simulink model "ThdRwLtStCalib"  (R2024b)
settings: Solver=FixedStepDiscrete  StartTime=0.0  StopTime=10.0  FixedStep=0.01  RelTol=1e-3
model workspace (MAT data in the model file):
  KeSMSwAcsMd6ThdRwLtStBkReclnUpwdDnwdPosMax_Val : Simulink.Parameter (value not decoded)
  KeSMSwAcsMd6ThdRwLtStBkReclnUpwdDnwdPosMin_Val : Simulink.Parameter (value not decoded)
  KeSMSwAcsMd6ThdRwLtStBkReclnUpwdDnwdPos_Val : Simulink.Parameter (value not decoded)
  KeSMSwAcsMd6ThdRwLtStCshnFldUpwdDnwdPosMax_Val : Simulink.Parameter (value not decoded)
  KeSMSwAcsMd6ThdRwLtStCshnFldUpwdDnwdPosMin_Val : Simulink.Parameter (value not decoded)
  KeSMSwAcsMd6ThdRwLtStCshnFldUpwdDnwdPos_Val : Simulink.Parameter (value not decoded)
  KeSMSwAcsMd6ThdRwLtStFrwdBkwdPosMax_Val : Simulink.Parameter (value not decoded)
  KeSMSwAcsMd6ThdRwLtStFrwdBkwdPosMin_Val : Simulink.Parameter (value not decoded)
  KeSMSwAcsMd6ThdRwLtStFrwdBkwdPos_Val : Simulink.Parameter (value not decoded)
symbols that are objects in the model workspace (value not decoded): KeSMSwAcsMd6ThdRwLtStBkReclnUpwdDnwdPos_Val, KeSMSwAcsMd6ThdRwLtStBkReclnUpwdDnwdPosMax_Val, KeSMSwAcsMd6ThdRwLtStBkReclnUpwdDnwdPosMin_Val, KeSMSwAcsMd6ThdRwLtStCshnFldUpwdDnwdPos_Val, KeSMSwAcsMd6ThdRwLtStCshnFldUpwdDnwdPosMax_Val, KeSMSwAcsMd6ThdRwLtStCshnFldUpwdDnwdPosMin_Val, KeSMSwAcsMd6ThdRwLtStFrwdBkwdPos_Val, KeSMSwAcsMd6ThdRwLtStFrwdBkwdPosMax_Val, KeSMSwAcsMd6ThdRwLtStFrwdBkwdPosMin_Val
undefined symbols (not defined in the file or in its folder): KeSMSw6sAcsEntryThdRwLtStBkReclnUpwdDnwdPos_Val, KeSMSw6sAcsEntryThdRwLtStBkReclnUpwdDnwdPosMax_Val, KeSMSw6sAcsEntryThdRwLtStBkReclnUpwdDnwdPosMin_Val, KeSMSw6sAcsEntryThdRwLtStCshnFldUpwdDnwdPos_Val, KeSMSw6sAcsEntryThdRwLtStCshnFldUpwdDnwdPosMax_Val, KeSMSw6sAcsEntryThdRwLtStCshnFldUpwdDnwdPosMin_Val, KeSMSw6sAcsEntryThdRwLtStFrwdBkwdPos_Val, KeSMSw6sAcsEntryThdRwLtStFrwdBkwdPosMax_Val, KeSMSw6sAcsEntryThdRwLtStFrwdBkwdPosMin_Val, KeSMSw6SAcsMd56ThdRwLtStBkReclnUpwdDnwdPos_Val, KeSMSw6SAcsMd56ThdRwLtStBkReclnUpwdDnwdPosMax_Val, KeSMSw6SAcsMd56ThdRwLtStBkReclnUpwdDnwdPosMin_Val, KeSMSw6SAcsMd56ThdRwLtStFrwdBkwdPos_Val, KeSMSw6SAcsMd56ThdRwLtStFrwdBkwdPosMax_Val, KeSMSw6SAcsMd56ThdRwLtStFrwdBkwdPosMin_Val, KeSMSw6sFamilyLMdThdRwLtStFrwdBkwdPos_Val, KeSMSw6sFamilyLMdThdRwLtStFrwdBkwdPosMax_Val, KeSMSw6sFamilyLMdThdRwLtStFrwdBkwdPosMin_Val, KeSMSw6sFamilyMdThdRwLtStFrwdBkwdPos_Val, KeSMSw6sFamilyMdThdRwLtStFrwdBkwdPosMax_Val, KeSMSw6sFamilyMdThdRwLtStFrwdBkwdPosMin_Val, KeSMSw6sLugThdRwLtStBkReclnUpwdDnwdPos_Val, KeSMSw6sLugThdRwLtStBkReclnUpwdDnwdPosMax_Val, KeSMSw6sLugThdRwLtStBkReclnUpwdDnwdPosMin_Val, KeSMSw6sLugThdRwLtStCshnFldUpwdDnwdPos_Val, KeSMSw6sLugThdRwLtStCshnFldUpwdDnwdPosMax_Val, KeSMSw6sLugThdRwLtStCshnFldUpwdDnwdPosMin_Val, KeSMSw6sVIPThdRwLtStBkReclnUpwdDnwdPos_Val, KeSMSw6sVIPThdRwLtStBkReclnUpwdDnwdPosMax_Val, KeSMSw6sVIPThdRwLtStBkReclnUpwdDnwdPosMin_Val, KeSMSw6sVIPThdRwLtStFrwdBkwdPos_Val, KeSMSw6sVIPThdRwLtStFrwdBkwdPosMax_Val, KeSMSw6sVIPThdRwLtStFrwdBkwdPosMin_Val, KeSMSwAcsEntryThdRwLtStBkReclnUpwdDnwdPos_Val, KeSMSwAcsEntryThdRwLtStBkReclnUpwdDnwdPosMax_Val, KeSMSwAcsEntryThdRwLtStBkReclnUpwdDnwdPosMin_Val, KeSMSwAcsEntryThdRwLtStCshnFldUpwdDnwdPos_Val, KeSMSwAcsEntryThdRwLtStCshnFldUpwdDnwdPosMax_Val, KeSMSwAcsEntryThdRwLtStCshnFldUpwdDnwdPosMin_Val, KeSMSwAcsEntryThdRwLtStFrwdBkwdPos_Val, KeSMSwAcsEntryThdRwLtStFrwdBkwdPosMax_Val, KeSMSwAcsEntryThdRwLtStFrwdBkwdPosMin_Val, KeSMSwAcsMd32ThdRwLtBkReclnUpwdDnwdPos_Val, KeSMSwAcsMd32ThdRwLtBkReclnUpwdDnwdPosMax_Val, KeSMSwAcsMd32ThdRwLtBkReclnUpwdDnwdPosMin_Val, KeSMSwAcsMd32ThdRwLtFldUpwdDnwdPos_Val, KeSMSwAcsMd32ThdRwLtFldUpwdDnwdPosMax_Val, KeSMSwAcsMd32ThdRwLtFldUpwdDnwdPosMin_Val, KeSMSwAcsMd56ThdRwLtStBkReclnUpwdDnwdPos_Val, KeSMSwAcsMd56ThdRwLtStBkReclnUpwdDnwdPosMax_Val, KeSMSwAcsMd56ThdRwLtStBkReclnUpwdDnwdPosMin_Val, KeSMSwAcsMd56ThdRwLtStCshnFldUpwdDnwdPos_Val, KeSMSwAcsMd56ThdRwLtStCshnFldUpwdDnwdPosMax_Val, KeSMSwAcsMd56ThdRwLtStCshnFldUpwdDnwdPosMin_Val, KeSMSwAcsMd56ThdRwLtStFrwdBkwdPos_Val, KeSMSwAcsMd56ThdRwLtStFrwdBkwdPosMax_Val, KeSMSwAcsMd56ThdRwLtStFrwdBkwdPosMin_Val, KeSMSwAcsMd57ThdRwLtStBkReclnUpwdDnwdPos_Val, KeSMSwAcsMd57ThdRwLtStBkReclnUpwdDnwdPosMax_Val, KeSMSwAcsMd57ThdRwLtStBkReclnUpwdDnwdPosMin_Val ... (+28)
libraries: TrgtPosSelcLib x20
(part 2 of 2)

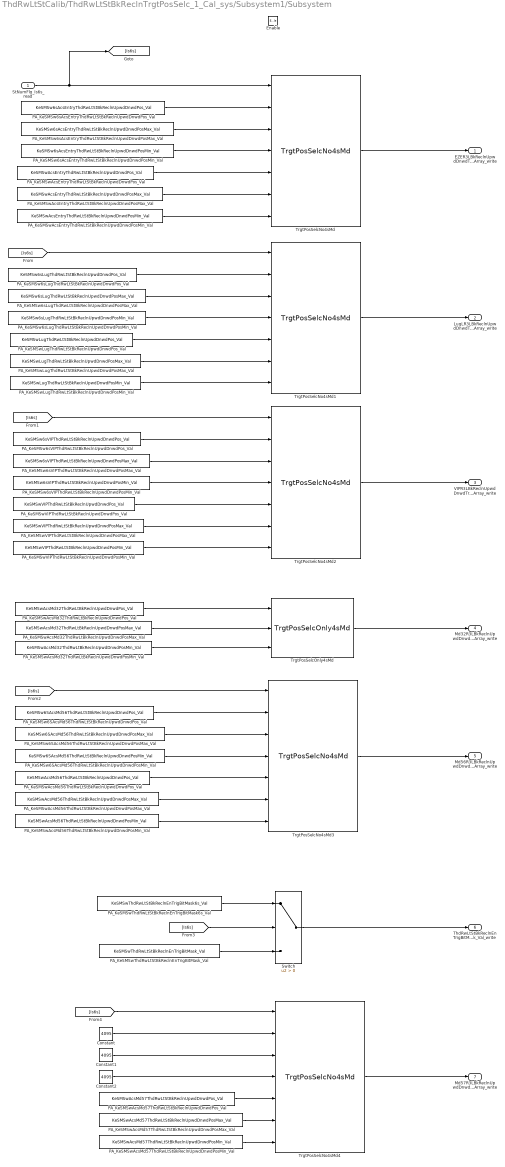
== system ThdRwLtStCalib/ThdRwLtStBkReclnTrgtPosSelc_1_Cal_sys/Subsystem1/Subsystem ==
  StNumFlg_Is6s_read : Inport
  Enable : EnablePort
  Constant : Constant  Value=4095  OutDataTypeStr=uint16
  Constant1 : Constant  Value=4095  OutDataTypeStr=uint16
  Constant2 : Constant  Value=4095  OutDataTypeStr=uint16
  PA_KeSMSw6SAcsMd56ThdRwLtStBkReclnUpwdDnwdPosMax_Val : Constant  Value=KeSMSw6SAcsMd56ThdRwLtStBkReclnUpwdDnwdPosMax_Val
  PA_KeSMSw6SAcsMd56ThdRwLtStBkReclnUpwdDnwdPosMin_Val : Constant  Value=KeSMSw6SAcsMd56ThdRwLtStBkReclnUpwdDnwdPosMin_Val
  PA_KeSMSw6SAcsMd56ThdRwLtStBkReclnUpwdDnwdPos_Val : Constant  Value=KeSMSw6SAcsMd56ThdRwLtStBkReclnUpwdDnwdPos_Val
  PA_KeSMSw6sAcsEntryThdRwLtStBkReclnUpwdDnwdPosMax_Val : Constant  Value=KeSMSw6sAcsEntryThdRwLtStBkReclnUpwdDnwdPosMax_Val
  PA_KeSMSw6sAcsEntryThdRwLtStBkReclnUpwdDnwdPosMin_Val : Constant  Value=KeSMSw6sAcsEntryThdRwLtStBkReclnUpwdDnwdPosMin_Val
  PA_KeSMSw6sAcsEntryThdRwLtStBkReclnUpwdDnwdPos_Val : Constant  Value=KeSMSw6sAcsEntryThdRwLtStBkReclnUpwdDnwdPos_Val
  PA_KeSMSw6sLugThdRwLtStBkReclnUpwdDnwdPosMax_Val : Constant  Value=KeSMSw6sLugThdRwLtStBkReclnUpwdDnwdPosMax_Val
  PA_KeSMSw6sLugThdRwLtStBkReclnUpwdDnwdPosMin_Val : Constant  Value=KeSMSw6sLugThdRwLtStBkReclnUpwdDnwdPosMin_Val
  PA_KeSMSw6sLugThdRwLtStBkReclnUpwdDnwdPos_Val : Constant  Value=KeSMSw6sLugThdRwLtStBkReclnUpwdDnwdPos_Val
  PA_KeSMSw6sVIPThdRwLtStBkReclnUpwdDnwdPosMax_Val : Constant  Value=KeSMSw6sVIPThdRwLtStBkReclnUpwdDnwdPosMax_Val
  PA_KeSMSw6sVIPThdRwLtStBkReclnUpwdDnwdPosMin_Val : Constant  Value=KeSMSw6sVIPThdRwLtStBkReclnUpwdDnwdPosMin_Val
  PA_KeSMSw6sVIPThdRwLtStBkReclnUpwdDnwdPos_Val : Constant  Value=KeSMSw6sVIPThdRwLtStBkReclnUpwdDnwdPos_Val
  PA_KeSMSwAcsEntryThdRwLtStBkReclnUpwdDnwdPosMax_Val : Constant  Value=KeSMSwAcsEntryThdRwLtStBkReclnUpwdDnwdPosMax_Val
  PA_KeSMSwAcsEntryThdRwLtStBkReclnUpwdDnwdPosMin_Val : Constant  Value=KeSMSwAcsEntryThdRwLtStBkReclnUpwdDnwdPosMin_Val
  PA_KeSMSwAcsEntryThdRwLtStBkReclnUpwdDnwdPos_Val : Constant  Value=KeSMSwAcsEntryThdRwLtStBkReclnUpwdDnwdPos_Val
  PA_KeSMSwAcsMd32ThdRwLtBkReclnUpwdDnwdPosMax_Val : Constant  Value=KeSMSwAcsMd32ThdRwLtBkReclnUpwdDnwdPosMax_Val
  PA_KeSMSwAcsMd32ThdRwLtBkReclnUpwdDnwdPosMin_Val : Constant  Value=KeSMSwAcsMd32ThdRwLtBkReclnUpwdDnwdPosMin_Val
  PA_KeSMSwAcsMd32ThdRwLtBkReclnUpwdDnwdPos_Val : Constant  Value=KeSMSwAcsMd32ThdRwLtBkReclnUpwdDnwdPos_Val
  PA_KeSMSwAcsMd56ThdRwLtStBkReclnUpwdDnwdPosMax_Val : Constant  Value=KeSMSwAcsMd56ThdRwLtStBkReclnUpwdDnwdPosMax_Val
  PA_KeSMSwAcsMd56ThdRwLtStBkReclnUpwdDnwdPosMin_Val : Constant  Value=KeSMSwAcsMd56ThdRwLtStBkReclnUpwdDnwdPosMin_Val
  PA_KeSMSwAcsMd56ThdRwLtStBkReclnUpwdDnwdPos_Val : Constant  Value=KeSMSwAcsMd56ThdRwLtStBkReclnUpwdDnwdPos_Val
  PA_KeSMSwAcsMd57ThdRwLtStBkReclnUpwdDnwdPosMax_Val : Constant  Value=KeSMSwAcsMd57ThdRwLtStBkReclnUpwdDnwdPosMax_Val
  PA_KeSMSwAcsMd57ThdRwLtStBkReclnUpwdDnwdPosMin_Val : Constant  Value=KeSMSwAcsMd57ThdRwLtStBkReclnUpwdDnwdPosMin_Val
  PA_KeSMSwAcsMd57ThdRwLtStBkReclnUpwdDnwdPos_Val : Constant  Value=KeSMSwAcsMd57ThdRwLtStBkReclnUpwdDnwdPos_Val
  PA_KeSMSwLugThdRwLtStBkReclnUpwdDnwdPosMax_Val : Constant  Value=KeSMSwLugThdRwLtStBkReclnUpwdDnwdPosMax_Val
  PA_KeSMSwLugThdRwLtStBkReclnUpwdDnwdPosMin_Val : Constant  Value=KeSMSwLugThdRwLtStBkReclnUpwdDnwdPosMin_Val
  PA_KeSMSwLugThdRwLtStBkReclnUpwdDnwdPos_Val : Constant  Value=KeSMSwLugThdRwLtStBkReclnUpwdDnwdPos_Val
  PA_KeSMSwThdRwLtStBkReclnEnTrigBitMask6s_Val : Constant  Value=KeSMSwThdRwLtStBkReclnEnTrigBitMask6s_Val
  PA_KeSMSwThdRwLtStBkReclnEnTrigBitMask_Val : Constant  Value=KeSMSwThdRwLtStBkReclnEnTrigBitMask_Val
  PA_KeSMSwVIPThdRwLtStBkReclnUpwdDnwdPosMax_Val : Constant  Value=KeSMSwVIPThdRwLtStBkReclnUpwdDnwdPosMax_Val
  PA_KeSMSwVIPThdRwLtStBkReclnUpwdDnwdPosMin_Val : Constant  Value=KeSMSwVIPThdRwLtStBkReclnUpwdDnwdPosMin_Val
  PA_KeSMSwVIPThdRwLtStBkReclnUpwdDnwdPos_Val : Constant  Value=KeSMSwVIPThdRwLtStBkReclnUpwdDnwdPos_Val
  Switch : Switch  Criteria=u2 > Threshold  SaturateOnIntegerOverflow=off  InputSameDT=off
  TrgtPosSelcNo4sMd{,1..4} (5 alike) : TrgtPosSelcLib/TrgtPosSelcNo4sMd  SystemSampleTime=-1  VariantActivationTime=update diagram  AllowFlexibleInterface=on  Latency=0  AutoFrameSizeCalculation=off
  TrgtPosSelcOnly4sMd : TrgtPosSelcLib/TrgtPosSelcOnly4sMd  SystemSampleTime=-1  VariantActivationTime=update diagram  AllowFlexibleInterface=on  Latency=0  AutoFrameSizeCalculation=off
  EZER3LBkReclnUpwdDnwdTrgtPosCalib_TrgtPosArray_write : Outport  VectorParamsAs1DForOutWhenUnconnected=off
      settings: EnsureOutportIsVirtual=on
  LugLR3LBkReclnUpwdDnwdTrgtPosCalib_TrgtPosArray_write : Outport  Port=2  VectorParamsAs1DForOutWhenUnconnected=off
      settings: EnsureOutportIsVirtual=on
  VIPR3LBkReclnUpwdDnwdTrgtPosCalib_TrgtPosArray_write : Outport  Port=3  VectorParamsAs1DForOutWhenUnconnected=off
      settings: EnsureOutportIsVirtual=on
  Md32R3LBkReclnUpwdDnwdTrgtPosCalib_TrgtPosArray_write : Outport  Port=4  VectorParamsAs1DForOutWhenUnconnected=off
      settings: EnsureOutportIsVirtual=on
  Md56R3LBkReclnUpwdDnwdTrgtPosCalib_TrgtPosArray_write : Outport  Port=5  VectorParamsAs1DForOutWhenUnconnected=off
      settings: EnsureOutportIsVirtual=on
  ThdRwLtStBkReclnEnTrigBitMask_Val_write : Outport  Port=6  VectorParamsAs1DForOutWhenUnconnected=off
      settings: EnsureOutportIsVirtual=on
  Md57R3LBkReclnUpwdDnwdTrgtPosCalib_TrgtPosArray_write : Outport  Port=7  VectorParamsAs1DForOutWhenUnconnected=off
      settings: EnsureOutportIsVirtual=on
  wires:
  StNumFlg_Is6s_read/1 -> [Is6s], TrgtPosSelcNo4sMd/1
  TrgtPosSelcNo4sMd1/1 -> LugLR3LBkReclnUpwdDnwdTrgtPosCalib_TrgtPosArray_write/1
  TrgtPosSelcNo4sMd2/1 -> VIPR3LBkReclnUpwdDnwdTrgtPosCalib_TrgtPosArray_write/1
  TrgtPosSelcNo4sMd/1 -> EZER3LBkReclnUpwdDnwdTrgtPosCalib_TrgtPosArray_write/1
  [Is6s] -> TrgtPosSelcNo4sMd1/1
  PA_KeSMSw6sAcsEntryThdRwLtStBkReclnUpwdDnwdPosMax_Val/1 -> TrgtPosSelcNo4sMd/3
  PA_KeSMSw6sAcsEntryThdRwLtStBkReclnUpwdDnwdPosMin_Val/1 -> TrgtPosSelcNo4sMd/4
  PA_KeSMSw6sAcsEntryThdRwLtStBkReclnUpwdDnwdPos_Val/1 -> TrgtPosSelcNo4sMd/2
  PA_KeSMSw6sLugThdRwLtStBkReclnUpwdDnwdPosMax_Val/1 -> TrgtPosSelcNo4sMd1/3
  PA_KeSMSw6sLugThdRwLtStBkReclnUpwdDnwdPos_Val/1 -> TrgtPosSelcNo4sMd1/2
  PA_KeSMSw6sLugThdRwLtStBkReclnUpwdDnwdPosMin_Val/1 -> TrgtPosSelcNo4sMd1/4
  [Is6s] -> TrgtPosSelcNo4sMd2/1
  PA_KeSMSw6sVIPThdRwLtStBkReclnUpwdDnwdPosMax_Val/1 -> TrgtPosSelcNo4sMd2/3
  PA_KeSMSw6sVIPThdRwLtStBkReclnUpwdDnwdPos_Val/1 -> TrgtPosSelcNo4sMd2/2
  PA_KeSMSw6sVIPThdRwLtStBkReclnUpwdDnwdPosMin_Val/1 -> TrgtPosSelcNo4sMd2/4
  PA_KeSMSwAcsEntryThdRwLtStBkReclnUpwdDnwdPosMax_Val/1 -> TrgtPosSelcNo4sMd/6
  PA_KeSMSwAcsEntryThdRwLtStBkReclnUpwdDnwdPosMin_Val/1 -> TrgtPosSelcNo4sMd/7
  PA_KeSMSwAcsEntryThdRwLtStBkReclnUpwdDnwdPos_Val/1 -> TrgtPosSelcNo4sMd/5
  PA_KeSMSwLugThdRwLtStBkReclnUpwdDnwdPosMax_Val/1 -> TrgtPosSelcNo4sMd1/6
  PA_KeSMSwLugThdRwLtStBkReclnUpwdDnwdPosMin_Val/1 -> TrgtPosSelcNo4sMd1/7
  PA_KeSMSwLugThdRwLtStBkReclnUpwdDnwdPos_Val/1 -> TrgtPosSelcNo4sMd1/5
  PA_KeSMSwVIPThdRwLtStBkReclnUpwdDnwdPosMax_Val/1 -> TrgtPosSelcNo4sMd2/6
  PA_KeSMSwVIPThdRwLtStBkReclnUpwdDnwdPos_Val/1 -> TrgtPosSelcNo4sMd2/5
  PA_KeSMSwVIPThdRwLtStBkReclnUpwdDnwdPosMin_Val/1 -> TrgtPosSelcNo4sMd2/7
  PA_KeSMSwAcsMd32ThdRwLtBkReclnUpwdDnwdPosMin_Val/1 -> TrgtPosSelcOnly4sMd/3
  PA_KeSMSwAcsMd32ThdRwLtBkReclnUpwdDnwdPosMax_Val/1 -> TrgtPosSelcOnly4sMd/2
  PA_KeSMSwAcsMd32ThdRwLtBkReclnUpwdDnwdPos_Val/1 -> TrgtPosSelcOnly4sMd/1
  TrgtPosSelcOnly4sMd/1 -> Md32R3LBkReclnUpwdDnwdTrgtPosCalib_TrgtPosArray_write/1
  [Is6s] -> TrgtPosSelcNo4sMd3/1
  PA_KeSMSw6SAcsMd56ThdRwLtStBkReclnUpwdDnwdPos_Val/1 -> TrgtPosSelcNo4sMd3/2
  PA_KeSMSw6SAcsMd56ThdRwLtStBkReclnUpwdDnwdPosMax_Val/1 -> TrgtPosSelcNo4sMd3/3
  PA_KeSMSw6SAcsMd56ThdRwLtStBkReclnUpwdDnwdPosMin_Val/1 -> TrgtPosSelcNo4sMd3/4
  PA_KeSMSwAcsMd56ThdRwLtStBkReclnUpwdDnwdPos_Val/1 -> TrgtPosSelcNo4sMd3/5
  PA_KeSMSwAcsMd56ThdRwLtStBkReclnUpwdDnwdPosMax_Val/1 -> TrgtPosSelcNo4sMd3/6
  PA_KeSMSwAcsMd56ThdRwLtStBkReclnUpwdDnwdPosMin_Val/1 -> TrgtPosSelcNo4sMd3/7
  TrgtPosSelcNo4sMd3/1 -> Md56R3LBkReclnUpwdDnwdTrgtPosCalib_TrgtPosArray_write/1
  PA_KeSMSwThdRwLtStBkReclnEnTrigBitMask6s_Val/1 -> Switch/1
  [Is6s] -> Switch/2
  PA_KeSMSwThdRwLtStBkReclnEnTrigBitMask_Val/1 -> Switch/3
  Switch/1 -> ThdRwLtStBkReclnEnTrigBitMask_Val_write/1
  [Is6s] -> TrgtPosSelcNo4sMd4/1
  PA_KeSMSwAcsMd57ThdRwLtStBkReclnUpwdDnwdPos_Val/1 -> TrgtPosSelcNo4sMd4/5
  PA_KeSMSwAcsMd57ThdRwLtStBkReclnUpwdDnwdPosMax_Val/1 -> TrgtPosSelcNo4sMd4/6
  PA_KeSMSwAcsMd57ThdRwLtStBkReclnUpwdDnwdPosMin_Val/1 -> TrgtPosSelcNo4sMd4/7
  Constant/1 -> TrgtPosSelcNo4sMd4/2
  Constant1/1 -> TrgtPosSelcNo4sMd4/3
  Constant2/1 -> TrgtPosSelcNo4sMd4/4
  TrgtPosSelcNo4sMd4/1 -> Md57R3LBkReclnUpwdDnwdTrgtPosCalib_TrgtPosArray_write/1

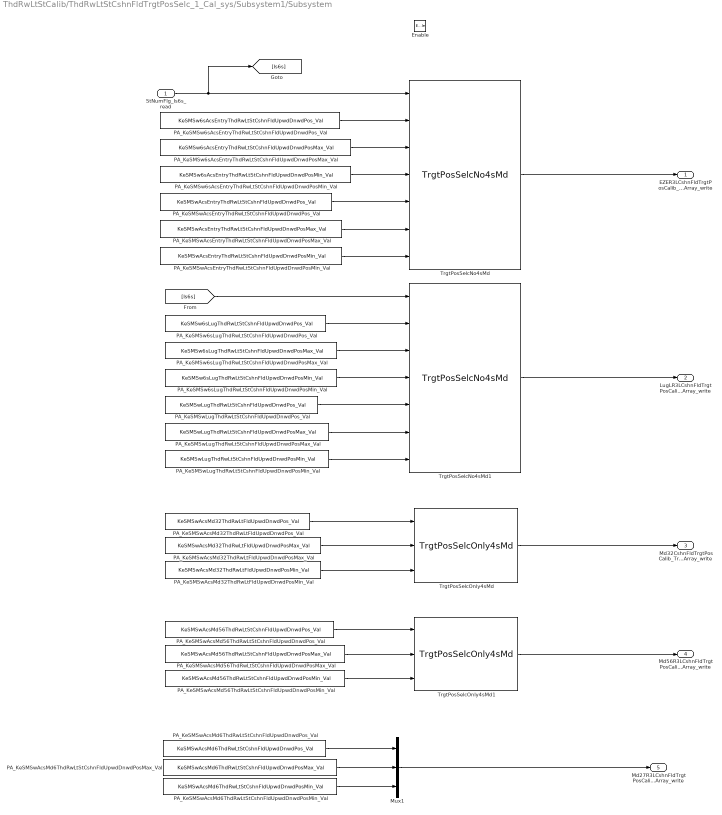
== system ThdRwLtStCalib/ThdRwLtStCshnFldTrgtPosSelc_1_Cal_sys/Subsystem1/Subsystem ==
  StNumFlg_Is6s_read : Inport
  Enable : EnablePort
  Mux1 : Mux  Inputs=3
  PA_KeSMSw6sAcsEntryThdRwLtStCshnFldUpwdDnwdPosMax_Val : Constant  Value=KeSMSw6sAcsEntryThdRwLtStCshnFldUpwdDnwdPosMax_Val
  PA_KeSMSw6sAcsEntryThdRwLtStCshnFldUpwdDnwdPosMin_Val : Constant  Value=KeSMSw6sAcsEntryThdRwLtStCshnFldUpwdDnwdPosMin_Val
  PA_KeSMSw6sAcsEntryThdRwLtStCshnFldUpwdDnwdPos_Val : Constant  Value=KeSMSw6sAcsEntryThdRwLtStCshnFldUpwdDnwdPos_Val
  PA_KeSMSw6sLugThdRwLtStCshnFldUpwdDnwdPosMax_Val : Constant  Value=KeSMSw6sLugThdRwLtStCshnFldUpwdDnwdPosMax_Val
  PA_KeSMSw6sLugThdRwLtStCshnFldUpwdDnwdPosMin_Val : Constant  Value=KeSMSw6sLugThdRwLtStCshnFldUpwdDnwdPosMin_Val
  PA_KeSMSw6sLugThdRwLtStCshnFldUpwdDnwdPos_Val : Constant  Value=KeSMSw6sLugThdRwLtStCshnFldUpwdDnwdPos_Val
  PA_KeSMSwAcsEntryThdRwLtStCshnFldUpwdDnwdPosMax_Val : Constant  Value=KeSMSwAcsEntryThdRwLtStCshnFldUpwdDnwdPosMax_Val
  PA_KeSMSwAcsEntryThdRwLtStCshnFldUpwdDnwdPosMin_Val : Constant  Value=KeSMSwAcsEntryThdRwLtStCshnFldUpwdDnwdPosMin_Val
  PA_KeSMSwAcsEntryThdRwLtStCshnFldUpwdDnwdPos_Val : Constant  Value=KeSMSwAcsEntryThdRwLtStCshnFldUpwdDnwdPos_Val
  PA_KeSMSwAcsMd32ThdRwLtFldUpwdDnwdPosMax_Val : Constant  Value=KeSMSwAcsMd32ThdRwLtFldUpwdDnwdPosMax_Val
  PA_KeSMSwAcsMd32ThdRwLtFldUpwdDnwdPosMin_Val : Constant  Value=KeSMSwAcsMd32ThdRwLtFldUpwdDnwdPosMin_Val
  PA_KeSMSwAcsMd32ThdRwLtFldUpwdDnwdPos_Val : Constant  Value=KeSMSwAcsMd32ThdRwLtFldUpwdDnwdPos_Val
  PA_KeSMSwAcsMd56ThdRwLtStCshnFldUpwdDnwdPosMax_Val : Constant  Value=KeSMSwAcsMd56ThdRwLtStCshnFldUpwdDnwdPosMax_Val
  PA_KeSMSwAcsMd56ThdRwLtStCshnFldUpwdDnwdPosMin_Val : Constant  Value=KeSMSwAcsMd56ThdRwLtStCshnFldUpwdDnwdPosMin_Val
  PA_KeSMSwAcsMd56ThdRwLtStCshnFldUpwdDnwdPos_Val : Constant  Value=KeSMSwAcsMd56ThdRwLtStCshnFldUpwdDnwdPos_Val
  PA_KeSMSwAcsMd6ThdRwLtStCshnFldUpwdDnwdPosMax_Val : Constant  Value=KeSMSwAcsMd6ThdRwLtStCshnFldUpwdDnwdPosMax_Val
  PA_KeSMSwAcsMd6ThdRwLtStCshnFldUpwdDnwdPosMin_Val : Constant  Value=KeSMSwAcsMd6ThdRwLtStCshnFldUpwdDnwdPosMin_Val
  PA_KeSMSwAcsMd6ThdRwLtStCshnFldUpwdDnwdPos_Val : Constant  Value=KeSMSwAcsMd6ThdRwLtStCshnFldUpwdDnwdPos_Val
  PA_KeSMSwLugThdRwLtStCshnFldUpwdDnwdPosMax_Val : Constant  Value=KeSMSwLugThdRwLtStCshnFldUpwdDnwdPosMax_Val
  PA_KeSMSwLugThdRwLtStCshnFldUpwdDnwdPosMin_Val : Constant  Value=KeSMSwLugThdRwLtStCshnFldUpwdDnwdPosMin_Val
  PA_KeSMSwLugThdRwLtStCshnFldUpwdDnwdPos_Val : Constant  Value=KeSMSwLugThdRwLtStCshnFldUpwdDnwdPos_Val
  TrgtPosSelcNo4sMd : TrgtPosSelcLib/TrgtPosSelcNo4sMd  SystemSampleTime=-1  VariantActivationTime=update diagram  AllowFlexibleInterface=on  Latency=0  AutoFrameSizeCalculation=off
  TrgtPosSelcNo4sMd1 : TrgtPosSelcLib/TrgtPosSelcNo4sMd  SystemSampleTime=-1  VariantActivationTime=update diagram  AllowFlexibleInterface=on  Latency=0  AutoFrameSizeCalculation=off
  TrgtPosSelcOnly4sMd : TrgtPosSelcLib/TrgtPosSelcOnly4sMd  SystemSampleTime=-1  VariantActivationTime=update diagram  AllowFlexibleInterface=on  Latency=0  AutoFrameSizeCalculation=off
  TrgtPosSelcOnly4sMd1 : TrgtPosSelcLib/TrgtPosSelcOnly4sMd  SystemSampleTime=-1  VariantActivationTime=update diagram  AllowFlexibleInterface=on  Latency=0  AutoFrameSizeCalculation=off
  EZER3LCshnFldTrgtPosCalib_TrgtPosArray_write : Outport  VectorParamsAs1DForOutWhenUnconnected=off
      settings: EnsureOutportIsVirtual=on
  LugLR3LCshnFldTrgtPosCalib_TrgtPosArray_write : Outport  Port=2  VectorParamsAs1DForOutWhenUnconnected=off
      settings: EnsureOutportIsVirtual=on
  Md32CshnFldTrgtPosCalib_TrgtPosArray_write : Outport  Port=3  VectorParamsAs1DForOutWhenUnconnected=off
      settings: EnsureOutportIsVirtual=on
  Md56R3LCshnFldTrgtPosCalib_TrgtPosArray_write : Outport  Port=4  VectorParamsAs1DForOutWhenUnconnected=off
      settings: EnsureOutportIsVirtual=on
  Md27R3LCshnFldTrgtPosCalib_TrgtPosArray_write : Outport  Port=5
  wires:
  StNumFlg_Is6s_read/1 -> [Is6s], TrgtPosSelcNo4sMd/1
  TrgtPosSelcNo4sMd1/1 -> LugLR3LCshnFldTrgtPosCalib_TrgtPosArray_write/1
  TrgtPosSelcNo4sMd/1 -> EZER3LCshnFldTrgtPosCalib_TrgtPosArray_write/1
  PA_KeSMSw6sAcsEntryThdRwLtStCshnFldUpwdDnwdPosMax_Val/1 -> TrgtPosSelcNo4sMd/3
  PA_KeSMSw6sAcsEntryThdRwLtStCshnFldUpwdDnwdPosMin_Val/1 -> TrgtPosSelcNo4sMd/4
  PA_KeSMSw6sAcsEntryThdRwLtStCshnFldUpwdDnwdPos_Val/1 -> TrgtPosSelcNo4sMd/2
  [Is6s] -> TrgtPosSelcNo4sMd1/1
  PA_KeSMSw6sLugThdRwLtStCshnFldUpwdDnwdPosMin_Val/1 -> TrgtPosSelcNo4sMd1/4
  PA_KeSMSw6sLugThdRwLtStCshnFldUpwdDnwdPosMax_Val/1 -> TrgtPosSelcNo4sMd1/3
  PA_KeSMSw6sLugThdRwLtStCshnFldUpwdDnwdPos_Val/1 -> TrgtPosSelcNo4sMd1/2
  PA_KeSMSwAcsEntryThdRwLtStCshnFldUpwdDnwdPosMax_Val/1 -> TrgtPosSelcNo4sMd/6
  PA_KeSMSwAcsEntryThdRwLtStCshnFldUpwdDnwdPosMin_Val/1 -> TrgtPosSelcNo4sMd/7
  PA_KeSMSwAcsEntryThdRwLtStCshnFldUpwdDnwdPos_Val/1 -> TrgtPosSelcNo4sMd/5
  PA_KeSMSwLugThdRwLtStCshnFldUpwdDnwdPosMax_Val/1 -> TrgtPosSelcNo4sMd1/6
  PA_KeSMSwLugThdRwLtStCshnFldUpwdDnwdPosMin_Val/1 -> TrgtPosSelcNo4sMd1/7
  PA_KeSMSwLugThdRwLtStCshnFldUpwdDnwdPos_Val/1 -> TrgtPosSelcNo4sMd1/5
  PA_KeSMSwAcsMd32ThdRwLtFldUpwdDnwdPos_Val/1 -> TrgtPosSelcOnly4sMd/1
  PA_KeSMSwAcsMd32ThdRwLtFldUpwdDnwdPosMax_Val/1 -> TrgtPosSelcOnly4sMd/2
  PA_KeSMSwAcsMd32ThdRwLtFldUpwdDnwdPosMin_Val/1 -> TrgtPosSelcOnly4sMd/3
  TrgtPosSelcOnly4sMd/1 -> Md32CshnFldTrgtPosCalib_TrgtPosArray_write/1
  TrgtPosSelcOnly4sMd1/1 -> Md56R3LCshnFldTrgtPosCalib_TrgtPosArray_write/1
  PA_KeSMSwAcsMd56ThdRwLtStCshnFldUpwdDnwdPos_Val/1 -> TrgtPosSelcOnly4sMd1/1
  PA_KeSMSwAcsMd56ThdRwLtStCshnFldUpwdDnwdPosMax_Val/1 -> TrgtPosSelcOnly4sMd1/2
  PA_KeSMSwAcsMd56ThdRwLtStCshnFldUpwdDnwdPosMin_Val/1 -> TrgtPosSelcOnly4sMd1/3
  PA_KeSMSwAcsMd6ThdRwLtStCshnFldUpwdDnwdPos_Val/1 -> Mux1/1
  PA_KeSMSwAcsMd6ThdRwLtStCshnFldUpwdDnwdPosMin_Val/1 -> Mux1/3
  PA_KeSMSwAcsMd6ThdRwLtStCshnFldUpwdDnwdPosMax_Val/1 -> Mux1/2
  Mux1/1 -> Md27R3LCshnFldTrgtPosCalib_TrgtPosArray_write/1

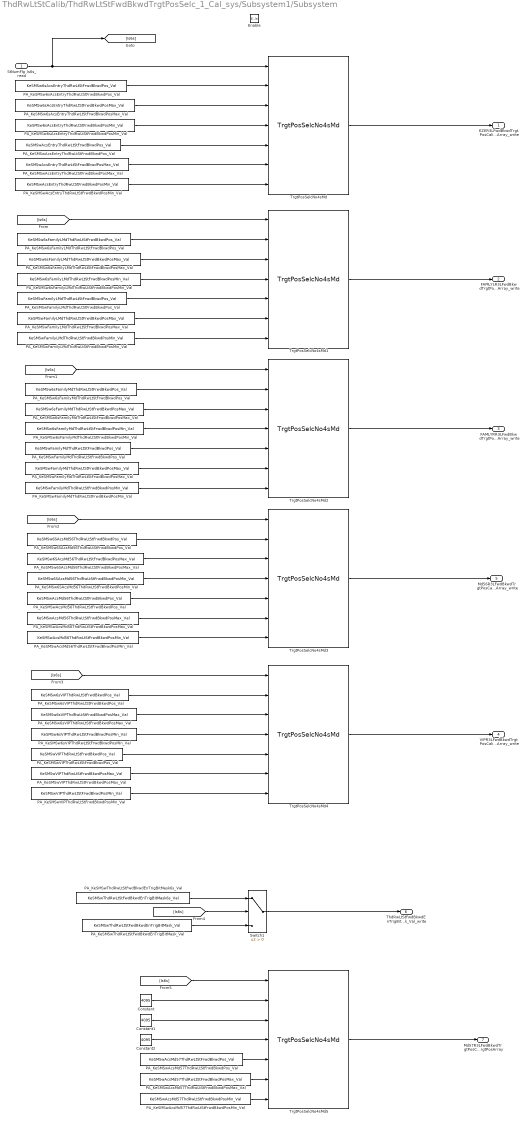
== system ThdRwLtStCalib/ThdRwLtStFwdBkwdTrgtPosSelc_1_Cal_sys/Subsystem1/Subsystem ==
  StNumFlg_Is6s_read : Inport
  Enable : EnablePort
  Constant : Constant  Value=4095  OutDataTypeStr=uint16
  Constant1 : Constant  Value=4095  OutDataTypeStr=uint16
  Constant2 : Constant  Value=4095  OutDataTypeStr=uint16
  PA_KeSMSw6SAcsMd56ThdRwLtStFrwdBkwdPosMax_Val : Constant  Value=KeSMSw6SAcsMd56ThdRwLtStFrwdBkwdPosMax_Val
  PA_KeSMSw6SAcsMd56ThdRwLtStFrwdBkwdPosMin_Val : Constant  Value=KeSMSw6SAcsMd56ThdRwLtStFrwdBkwdPosMin_Val
  PA_KeSMSw6SAcsMd56ThdRwLtStFrwdBkwdPos_Val : Constant  Value=KeSMSw6SAcsMd56ThdRwLtStFrwdBkwdPos_Val
  PA_KeSMSw6sAcsEntryThdRwLtStFrwdBkwdPosMax_Val : Constant  Value=KeSMSw6sAcsEntryThdRwLtStFrwdBkwdPosMax_Val
  PA_KeSMSw6sAcsEntryThdRwLtStFrwdBkwdPosMin_Val : Constant  Value=KeSMSw6sAcsEntryThdRwLtStFrwdBkwdPosMin_Val
  PA_KeSMSw6sAcsEntryThdRwLtStFrwdBkwdPos_Val : Constant  Value=KeSMSw6sAcsEntryThdRwLtStFrwdBkwdPos_Val
  PA_KeSMSw6sFamilyLMdThdRwLtStFrwdBkwdPosMax_Val : Constant  Value=KeSMSw6sFamilyLMdThdRwLtStFrwdBkwdPosMax_Val
  PA_KeSMSw6sFamilyLMdThdRwLtStFrwdBkwdPosMin_Val : Constant  Value=KeSMSw6sFamilyLMdThdRwLtStFrwdBkwdPosMin_Val
  PA_KeSMSw6sFamilyLMdThdRwLtStFrwdBkwdPos_Val : Constant  Value=KeSMSw6sFamilyLMdThdRwLtStFrwdBkwdPos_Val
  PA_KeSMSw6sFamilyMdThdRwLtStFrwdBkwdPosMax_Val : Constant  Value=KeSMSw6sFamilyMdThdRwLtStFrwdBkwdPosMax_Val
  PA_KeSMSw6sFamilyMdThdRwLtStFrwdBkwdPosMin_Val : Constant  Value=KeSMSw6sFamilyMdThdRwLtStFrwdBkwdPosMin_Val
  PA_KeSMSw6sFamilyMdThdRwLtStFrwdBkwdPos_Val : Constant  Value=KeSMSw6sFamilyMdThdRwLtStFrwdBkwdPos_Val
  PA_KeSMSw6sVIPThdRwLtStFrwdBkwdPosMax_Val : Constant  Value=KeSMSw6sVIPThdRwLtStFrwdBkwdPosMax_Val
  PA_KeSMSw6sVIPThdRwLtStFrwdBkwdPosMin_Val : Constant  Value=KeSMSw6sVIPThdRwLtStFrwdBkwdPosMin_Val
  PA_KeSMSw6sVIPThdRwLtStFrwdBkwdPos_Val : Constant  Value=KeSMSw6sVIPThdRwLtStFrwdBkwdPos_Val
  PA_KeSMSwAcsEntryThdRwLtStFrwdBkwdPosMax_Val : Constant  Value=KeSMSwAcsEntryThdRwLtStFrwdBkwdPosMax_Val
  PA_KeSMSwAcsEntryThdRwLtStFrwdBkwdPosMin_Val : Constant  Value=KeSMSwAcsEntryThdRwLtStFrwdBkwdPosMin_Val
  PA_KeSMSwAcsEntryThdRwLtStFrwdBkwdPos_Val : Constant  Value=KeSMSwAcsEntryThdRwLtStFrwdBkwdPos_Val
  PA_KeSMSwAcsMd56ThdRwLtStFrwdBkwdPosMax_Val : Constant  Value=KeSMSwAcsMd56ThdRwLtStFrwdBkwdPosMax_Val
  PA_KeSMSwAcsMd56ThdRwLtStFrwdBkwdPosMin_Val : Constant  Value=KeSMSwAcsMd56ThdRwLtStFrwdBkwdPosMin_Val
  PA_KeSMSwAcsMd56ThdRwLtStFrwdBkwdPos_Val : Constant  Value=KeSMSwAcsMd56ThdRwLtStFrwdBkwdPos_Val
  PA_KeSMSwAcsMd57ThdRwLtStFrwdBkwdPosMax_Val : Constant  Value=KeSMSwAcsMd57ThdRwLtStFrwdBkwdPosMax_Val
  PA_KeSMSwAcsMd57ThdRwLtStFrwdBkwdPosMin_Val : Constant  Value=KeSMSwAcsMd57ThdRwLtStFrwdBkwdPosMin_Val
  PA_KeSMSwAcsMd57ThdRwLtStFrwdBkwdPos_Val : Constant  Value=KeSMSwAcsMd57ThdRwLtStFrwdBkwdPos_Val
  PA_KeSMSwFamilyLMdThdRwLtStFrwdBkwdPosMax_Val : Constant  Value=KeSMSwFamilyLMdThdRwLtStFrwdBkwdPosMax_Val
  PA_KeSMSwFamilyLMdThdRwLtStFrwdBkwdPosMin_Val : Constant  Value=KeSMSwFamilyLMdThdRwLtStFrwdBkwdPosMin_Val
  PA_KeSMSwFamilyLMdThdRwLtStFrwdBkwdPos_Val : Constant  Value=KeSMSwFamilyLMdThdRwLtStFrwdBkwdPos_Val
  PA_KeSMSwFamilyMdThdRwLtStFrwdBkwdPosMax_Val : Constant  Value=KeSMSwFamilyMdThdRwLtStFrwdBkwdPosMax_Val
  PA_KeSMSwFamilyMdThdRwLtStFrwdBkwdPosMin_Val : Constant  Value=KeSMSwFamilyMdThdRwLtStFrwdBkwdPosMin_Val
  PA_KeSMSwFamilyMdThdRwLtStFrwdBkwdPos_Val : Constant  Value=KeSMSwFamilyMdThdRwLtStFrwdBkwdPos_Val
  PA_KeSMSwThdRwLtStFwdBkwdEnTrigBitMask6s_Val : Constant  Value=KeSMSwThdRwLtStFwdBkwdEnTrigBitMask6s_Val
  PA_KeSMSwThdRwLtStFwdBkwdEnTrigBitMask_Val : Constant  Value=KeSMSwThdRwLtStFwdBkwdEnTrigBitMask_Val
  PA_KeSMSwVIPThdRwLtStFrwdBkwdPosMax_Val : Constant  Value=KeSMSwVIPThdRwLtStFrwdBkwdPosMax_Val
  PA_KeSMSwVIPThdRwLtStFrwdBkwdPosMin_Val : Constant  Value=KeSMSwVIPThdRwLtStFrwdBkwdPosMin_Val
  PA_KeSMSwVIPThdRwLtStFrwdBkwdPos_Val : Constant  Value=KeSMSwVIPThdRwLtStFrwdBkwdPos_Val
  Switch1 : Switch  Criteria=u2 > Threshold  SaturateOnIntegerOverflow=off  InputSameDT=off
  TrgtPosSelcNo4sMd{,1..5} (6 alike) : TrgtPosSelcLib/TrgtPosSelcNo4sMd  SystemSampleTime=-1  VariantActivationTime=update diagram  AllowFlexibleInterface=on  Latency=0  AutoFrameSizeCalculation=off
  EZER3LFwdBkwdTrgtPosCalib_TrgtPosArray_write : Outport  VectorParamsAs1DForOutWhenUnconnected=off
      settings: EnsureOutportIsVirtual=on
  FAMLYLR3LFwdBkwdTrgtPosCalib_TrgtPosArray_write : Outport  Port=2  VectorParamsAs1DForOutWhenUnconnected=off
      settings: EnsureOutportIsVirtual=on
  FAMLYRR3LFwdBkwdTrgtPosCalib_TrgtPosArray_write : Outport  Port=3  VectorParamsAs1DForOutWhenUnconnected=off
      settings: EnsureOutportIsVirtual=on
  VIPR3LFwdBkwdTrgtPosCalib_TrgtPosArray_write : Outport  Port=4  VectorParamsAs1DForOutWhenUnconnected=off
      settings: EnsureOutportIsVirtual=on
  Md56R3LFwdBkwdTrgtPosCalib_TrgtPosArray_write : Outport  Port=5  VectorParamsAs1DForOutWhenUnconnected=off
      settings: EnsureOutportIsVirtual=on
  ThdRwLtStFwdBkwdEnTrigBitMask_Val_write : Outport  Port=6  VectorParamsAs1DForOutWhenUnconnected=off
      settings: EnsureOutportIsVirtual=on
  Md57R3LFwdBkwdTrgtPosCalib_TrgtPosArray : Outport  Description=|  Port=7  OutDataTypeStr=uint16  PortDimensions=3  VectorParamsAs1DForOutWhenUnconnected=off
      | 0:Pos
      | 1:Max
      | 2:Min
  wires:
  StNumFlg_Is6s_read/1 -> [Is6s], TrgtPosSelcNo4sMd/1
  TrgtPosSelcNo4sMd/1 -> EZER3LFwdBkwdTrgtPosCalib_TrgtPosArray_write/1
  TrgtPosSelcNo4sMd1/1 -> FAMLYLR3LFwdBkwdTrgtPosCalib_TrgtPosArray_write/1
  TrgtPosSelcNo4sMd2/1 -> FAMLYRR3LFwdBkwdTrgtPosCalib_TrgtPosArray_write/1
  TrgtPosSelcNo4sMd4/1 -> VIPR3LFwdBkwdTrgtPosCalib_TrgtPosArray_write/1
  PA_KeSMSw6sAcsEntryThdRwLtStFrwdBkwdPosMax_Val/1 -> TrgtPosSelcNo4sMd/3
  PA_KeSMSw6sAcsEntryThdRwLtStFrwdBkwdPosMin_Val/1 -> TrgtPosSelcNo4sMd/4
  PA_KeSMSw6sAcsEntryThdRwLtStFrwdBkwdPos_Val/1 -> TrgtPosSelcNo4sMd/2
  [Is6s] -> TrgtPosSelcNo4sMd1/1
  PA_KeSMSw6sFamilyLMdThdRwLtStFrwdBkwdPosMax_Val/1 -> TrgtPosSelcNo4sMd1/3
  PA_KeSMSw6sFamilyLMdThdRwLtStFrwdBkwdPosMin_Val/1 -> TrgtPosSelcNo4sMd1/4
  PA_KeSMSw6sFamilyLMdThdRwLtStFrwdBkwdPos_Val/1 -> TrgtPosSelcNo4sMd1/2
  [Is6s] -> TrgtPosSelcNo4sMd2/1
  [Is6s] -> TrgtPosSelcNo4sMd4/1
  PA_KeSMSw6sFamilyMdThdRwLtStFrwdBkwdPosMax_Val/1 -> TrgtPosSelcNo4sMd2/3
  PA_KeSMSw6sFamilyMdThdRwLtStFrwdBkwdPosMin_Val/1 -> TrgtPosSelcNo4sMd2/4
  PA_KeSMSw6sFamilyMdThdRwLtStFrwdBkwdPos_Val/1 -> TrgtPosSelcNo4sMd2/2
  PA_KeSMSw6sVIPThdRwLtStFrwdBkwdPosMax_Val/1 -> TrgtPosSelcNo4sMd4/3
  PA_KeSMSw6sVIPThdRwLtStFrwdBkwdPos_Val/1 -> TrgtPosSelcNo4sMd4/2
  PA_KeSMSw6sVIPThdRwLtStFrwdBkwdPosMin_Val/1 -> TrgtPosSelcNo4sMd4/4
  PA_KeSMSwAcsEntryThdRwLtStFrwdBkwdPosMax_Val/1 -> TrgtPosSelcNo4sMd/6
  PA_KeSMSwAcsEntryThdRwLtStFrwdBkwdPos_Val/1 -> TrgtPosSelcNo4sMd/5
  PA_KeSMSwAcsEntryThdRwLtStFrwdBkwdPosMin_Val/1 -> TrgtPosSelcNo4sMd/7
  PA_KeSMSwFamilyLMdThdRwLtStFrwdBkwdPosMax_Val/1 -> TrgtPosSelcNo4sMd1/6
  PA_KeSMSwFamilyLMdThdRwLtStFrwdBkwdPosMin_Val/1 -> TrgtPosSelcNo4sMd1/7
  PA_KeSMSwFamilyLMdThdRwLtStFrwdBkwdPos_Val/1 -> TrgtPosSelcNo4sMd1/5
  PA_KeSMSwFamilyMdThdRwLtStFrwdBkwdPosMax_Val/1 -> TrgtPosSelcNo4sMd2/6
  PA_KeSMSwFamilyMdThdRwLtStFrwdBkwdPosMin_Val/1 -> TrgtPosSelcNo4sMd2/7
  PA_KeSMSwFamilyMdThdRwLtStFrwdBkwdPos_Val/1 -> TrgtPosSelcNo4sMd2/5
  PA_KeSMSwVIPThdRwLtStFrwdBkwdPosMax_Val/1 -> TrgtPosSelcNo4sMd4/6
  PA_KeSMSwVIPThdRwLtStFrwdBkwdPos_Val/1 -> TrgtPosSelcNo4sMd4/5
  PA_KeSMSwVIPThdRwLtStFrwdBkwdPosMin_Val/1 -> TrgtPosSelcNo4sMd4/7
  PA_KeSMSwAcsMd56ThdRwLtStFrwdBkwdPos_Val/1 -> TrgtPosSelcNo4sMd3/5
  PA_KeSMSwAcsMd56ThdRwLtStFrwdBkwdPosMin_Val/1 -> TrgtPosSelcNo4sMd3/7
  PA_KeSMSwAcsMd56ThdRwLtStFrwdBkwdPosMax_Val/1 -> TrgtPosSelcNo4sMd3/6
  PA_KeSMSw6SAcsMd56ThdRwLtStFrwdBkwdPos_Val/1 -> TrgtPosSelcNo4sMd3/2
  PA_KeSMSw6SAcsMd56ThdRwLtStFrwdBkwdPosMin_Val/1 -> TrgtPosSelcNo4sMd3/4
  PA_KeSMSw6SAcsMd56ThdRwLtStFrwdBkwdPosMax_Val/1 -> TrgtPosSelcNo4sMd3/3
  [Is6s] -> TrgtPosSelcNo4sMd3/1
  TrgtPosSelcNo4sMd3/1 -> Md56R3LFwdBkwdTrgtPosCalib_TrgtPosArray_write/1
  PA_KeSMSwThdRwLtStFwdBkwdEnTrigBitMask6s_Val/1 -> Switch1/1
  [Is6s] -> Switch1/2
  Switch1/1 -> ThdRwLtStFwdBkwdEnTrigBitMask_Val_write/1
  PA_KeSMSwThdRwLtStFwdBkwdEnTrigBitMask_Val/1 -> Switch1/3
  TrgtPosSelcNo4sMd5/1 -> Md57R3LFwdBkwdTrgtPosCalib_TrgtPosArray/1
  [Is6s] -> TrgtPosSelcNo4sMd5/1
  Constant/1 -> TrgtPosSelcNo4sMd5/2
  Constant1/1 -> TrgtPosSelcNo4sMd5/3
  Constant2/1 -> TrgtPosSelcNo4sMd5/4
  PA_KeSMSwAcsMd57ThdRwLtStFrwdBkwdPos_Val/1 -> TrgtPosSelcNo4sMd5/5
  PA_KeSMSwAcsMd57ThdRwLtStFrwdBkwdPosMin_Val/1 -> TrgtPosSelcNo4sMd5/7
  PA_KeSMSwAcsMd57ThdRwLtStFrwdBkwdPosMax_Val/1 -> TrgtPosSelcNo4sMd5/6
